simulink model "model_relay"  (R2016b)
settings: Solver=VariableStepAuto  StartTime=0.0  StopTime=10  RelTol=1e-3
undefined symbols (not defined in the file or in its folder): Capacitor, Start
libraries: powerlib x4
settings Model: Creator=Chandan  LastModifiedBy=Chandan

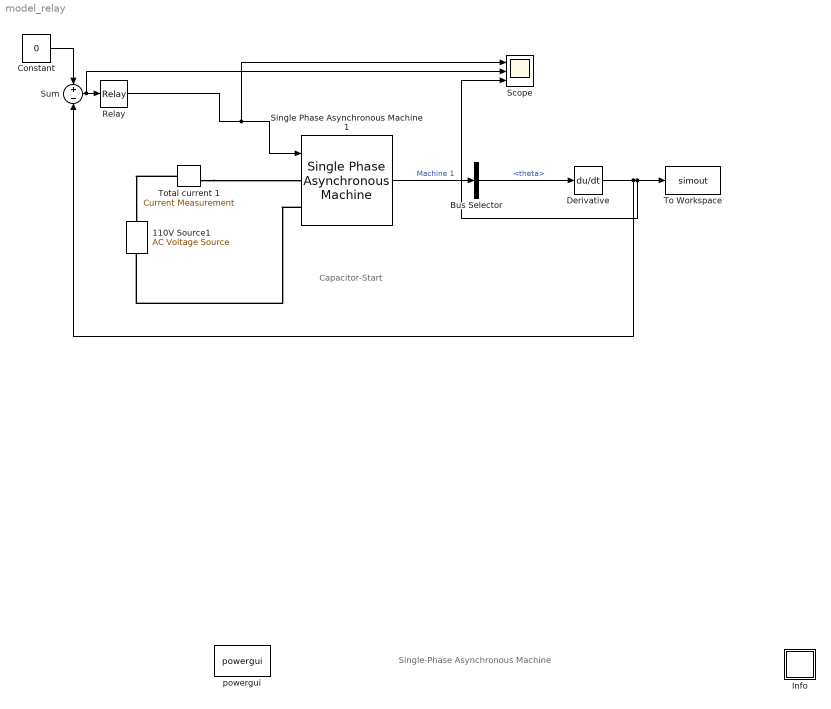
== system model_relay ==
  note: Capacitor-Start
  note: Single-Phase Asynchronous Machine
  110V Source1 : powerlib/Electrical Sources/AC Voltage Source  Amplitude=220*sqrt(2)  Phase=90  Frequency=60  SampleTime=0  Measurements=Voltage  BusType=swing  Pref=10e3  Qref=0  Qmin=-inf  Qmax=+inf
  Bus Selector : BusSelector  OutputSignals=theta
  Constant : Constant  Value=0
  Derivative : Derivative
  Info : Subsystem
      settings: OpenFcn=showdemo(bdroot(gcb))
      mask Display: disp('?')
  Relay : Relay  OnSwitchValue=-185  OffSwitchValue=-187  OnOutputValue=5
  Scope : Scope  NumInputPorts=3
  Single Phase Asynchronous Machine 1 : powerlib/Machines/Single Phase Asynchronous Machine  MechanicalLoad=Torque Tm  UNITS=SI  MachineType=Capacitor-Start  MeasurementBus=on  NominalParameters="[ .25*746  110  60]"  MainWindingStator="[2.02  7.4e-3]"  MainWindingRotor="[4.12  5.6e-3]"  MutualInductance=0.177  AuxiliaryWinding=[7.14 8.54e-3]  Mechanical=[0.0146 0 2 1.18]  CapacitorStart="[2.15  255e-6]"  CapacitorRun=[0.04624 1592]  DisconnectionSpeed=75  InitialSpeed=0  DataType=SI  TsPowergui=0  TsBlock=-1
  Sum : Sum  Inputs=+-
  To Workspace : ToWorkspace  VariableName=simout  SaveFormat=Timeseries  SampleTime=-1
  Total current 1 : powerlib/Measurements/Current Measurement  PhasorSimulation=off  OutputType=Complex  PSBequivalent=0
  powergui : powerlib/powergui  SimulationMode=Continuous  SolverType=Tustin  SampleTime=1e-5  frequency=60  SPID=on  DisableSnubberDevices=off  DisableRonSwitches=off  DisableVfSwitches=off  SwTol=0  DisplayEquations=off  Interpol=off  ExternalGateDelay=off  methode=off  Ts=0  FunctionMessages=off  echomessages=off  HookPort=off  EnableUseOfTLC=off  x0status=blocks  frequencyindice=60  Pbase=100e6  ErrMax=1e-4  Iterations=50  UnitsV=kV  UnitsW=MW  buscounter=0  RestoreLinks=warning  ResistiveCurrentMeasurement=off  Frange=[0:2:500]  Ylog=off  Xlog=on  ShowGrid=off  save=off  variable=ZData  structure=0  ZoomFFT=on  StartTime=0.0  cycles=1  DisplayStyle=1  fundamental=60  FreqAxis=off  MaxFrequency=1000  frequencyindicesteady=1  RmsSteady=1  display=off
  wires:
  Bus Selector/1 -> Derivative/1  "<theta>"
  Relay/1 -> Scope/1, Single Phase Asynchronous Machine 1/1
  Single Phase Asynchronous Machine 1/1 -> Bus Selector/1  "Machine 1"
  Constant/1 -> Sum/1
  Sum/1 -> Scope/2, Relay/1
  Derivative/1 -> Sum/2, Scope/3, To Workspace/1
  connections:
  Total current 1/RConn1 -- Single Phase Asynchronous Machine 1/LConn1
  Single Phase Asynchronous Machine 1/LConn2 -- 110V Source1/LConn1
  Total current 1/LConn1 -- 110V Source1/RConn1

== system model_relay/Info ==
